simulink model "model_tou_muhsinov_p"  (R2021b)
settings: Solver=VariableStepAuto  StartTime=0.0  StopTime=2  RelTol=1e-6
model workspace (MAT data in the model file):
  G = [1.4 1.5 0.6 0.6 0.6 0.6 0.2 0.2 0.2 1.3 1.3 0.2 0.2 1.3 1.3 0.2 0.2 0.2 1.3 1.3 0.2 1.3 1.3 1.3 0.2 0.2 0.2 1.3 1.3 1.3 0.2 0.2]
values from neighbouring files (symbols this model uses):
  A = [-1*(1/t_p+1/t_retention), 1/t_release,2/t_ion; 1/t_retention, -1/t_release, 0; 1/(2*t_p), 0, -1*(1/t_pump+1/t_ion)]    [gui_tau_pump.m]
  B = [0;0;1]    [gui_tau_pump.m]
  C = [1,0,0; 0, 0, 1]    [gui_tau_pump.m]
  D = [0; 0];assignin("base","B", B)    [gui_tau_pump.m]
libraries: simulink x2
settings Model: Creator=pavlov  LastModifiedBy=pavlov

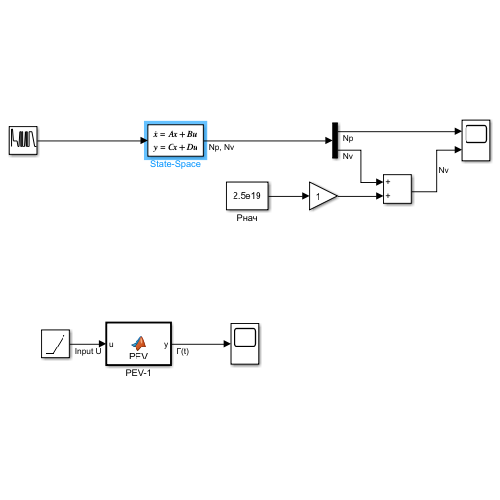
[thumbnail: Simulink's stored preview of the top-level diagram]
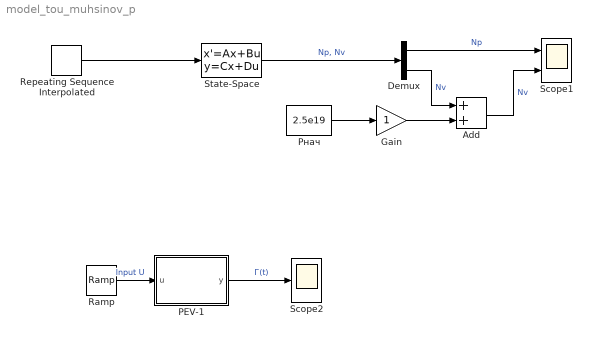
== system model_tou_muhsinov_p ==
  Add : Sum
  Demux : Demux  Outputs=2
  Gain : Gain
  PEV-1 : MATLAB Function  TreatAsAtomicUnit=on
  Pнач : Constant  Value=2.5e19
  Ramp : simulink/Sources/Ramp  slope=100  start=0  InitialOutput=0
  Repeating Sequence Interpolated : simulink/Sources/Repeating Sequence Interpolated  OutValues=[1.4 1.5 0.6 0.6 0.6 0.6 0.2 0.2 0.2 1.3 1.3 0.2 0.2 1.3 1.3 0.2 0.2 0.2 1.3 1.3 0.2 1.3 1.3 1.3 0.2 0.2 0.2 1.3 1.3 1.3 0.2 0.2]*1e21.'  TimeValues=[0 0.1 0.2 0.3 0.4 0.45 0.5 0.55, 0.6, 0.7 0.72 0.76 0.8 0.85 0.9 0.92 1 1.05 1.1 1.13 1.15 1.18 1.2 1.22 1.24 1.3 1.37 1.4 1.5 1.6 1.8 2.0].'  LookUpMeth=Interpolation-Use End Values  tsamp=0.01  OutMin=[]  OutMax=[]  OutDataTypeStr=double  OutputDataTypeScalingMode=double  OutDataType=fixdt(0,8)  OutScaling=2^-10
  Scope1 : Scope  NumInputPorts=2
  Scope2 : Scope
  State-Space : StateSpace  A=A  B=B  C=C  D=D  InitialCondition=0
  wires:
  Ramp/1 -> PEV-1/1(u)  "Input U"
  PEV-1/1(y) -> Scope2/1  "Г(t)"
  State-Space/1 -> Demux/1  "Np, Nv"
  Demux/1 -> Scope1/1  "Np"
  Pнач/1 -> Gain/1
  Gain/1 -> Add/2
  Repeating Sequence Interpolated/1 -> State-Space/1
  Demux/2 -> Add/1  "Nv"
  Add/1 -> Scope1/2  "Nv"

== matlab function model_tou_muhsinov_p/PEV-1 ==
  data: u input; y output
function y = PEV(u)
    y_vals = [0, 18, 28, 42, 62, 80, 100, 123, 154, 180, 200, 232, 259, 280, 300, 323, 346, 360, 400, 433, 450, 478, 500, 538, 552, 580, 600, 635, 668, 700, 729, 750, 770, 800, 839, 870, 900, 930, 958, 988, 1000, 1050, 1100];
    x_vals = [20, 32, 35, 40, 44.8, 48.2, 50, 52.2, 54.8, 56.5, 57.5, 60, 61.7, 62.8, 63.9, 65, 66.1, 67.5, 70, 71, 72, 74, 75, 76.5, 78, 80, 82, 83, 85, 87, 88, 90, 90.8, 91.8, 93, 94.5, 96.2, 97.2, 98, 98.2, 98.5, 98.8, 99];
    Gase = interp1(x_vals, y_vals, u);
    y = Gase;
end
